simulink model "sistema_plantilla"  (R2024b)
settings: Solver=VariableStepAuto  StartTime=0.0  StopTime=10.0  RelTol=1e-3
settings Model: Creator=juanb  LastModifiedBy=juanb

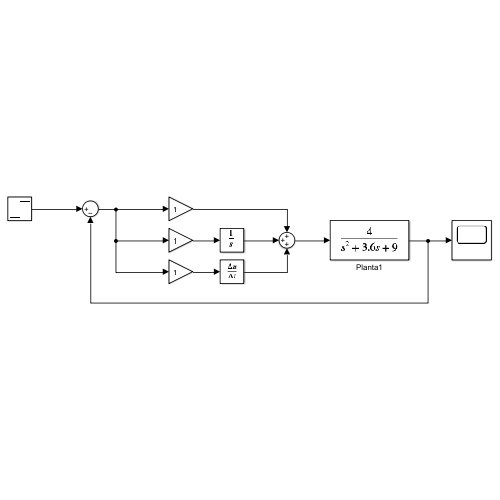
[thumbnail: Simulink's stored preview of the top-level diagram]
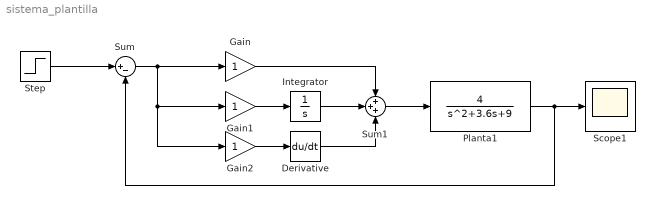
== system sistema_plantilla ==
  Derivative : Derivative
  Gain : Gain
  Gain1 : Gain
  Gain2 : Gain
  Integrator : Integrator
  Planta1 : TransferFcn  Numerator=[4]  Denominator=[1 3.6 9]
  Scope1 : Scope
  Step : Step  SampleTime=0
  Sum : Sum  Inputs=|+-
  Sum1 : Sum  Inputs=+++
  wires:
  Step/1 -> Sum/1
  Sum/1 -> Gain1/1, Gain2/1, Gain/1
  Gain2/1 -> Derivative/1
  Gain1/1 -> Integrator/1
  Gain/1 -> Sum1/1
  Integrator/1 -> Sum1/2
  Derivative/1 -> Sum1/3
  Sum1/1 -> Planta1/1
  Planta1/1 -> Sum/2, Scope1/1
